simulink model "sim_notch440"  (R2021a)
settings: Solver=FixedStepDiscrete  StartTime=0.0  StopTime=3.9  FixedStep=6.25e-5  RelTol=1e-3
libraries: dspvision x1, simulink x1
settings Model: Creator=ricar  LastModifiedBy=rodri
settings SolverCC: AlgebraicLoopSolver=TrustRegion
settings DebuggingCC: SFMachineParentedDataDiag=warning

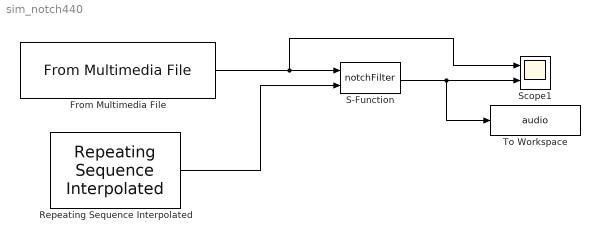
== system sim_notch440 ==
  From Multimedia File : dspvision/From Multimedia File  inputFilename=C:\Users\rodri\Desktop\Semestre_11\ELO314_Lab-DSP\Lab-DSP\lab3dsp_G6_Graves_Mardones\labC\sources\s-function_notch2\alternate_tones_16_16.wav  readRange=[1 Inf]  loop=on  numPlays=inf  outputStreams=Audio only  videoDataType=single  audioDataType=double  inheritSampleTime=on  userDefinedSampleTime=1/30  noAudioOutput=off  isIntensityVideo=off  fourcc=RGB  colorVideoFormat=Separate color signals  outputEOF=off  dataOrg=Column-major  audioFrameSize=1  computeAudioFrameSize=off  outSamplingMode=Sample based
  Repeating Sequence Interpolated : simulink/Sources/Repeating Sequence Interpolated  OutValues=[440 440 880 880].'  TimeValues=[0 1 3 4].'  LookUpMeth=Interpolation-Use End Values  tsamp=0.01  OutMin=[]  OutMax=[]  OutDataTypeStr=double  OutputDataTypeScalingMode=double  OutDataType=fixdt(0,8)  OutScaling=2^-10
  S-Function : S-Function  FunctionName=notchFilter  SFunctionDeploymentMode=off  EnableBusSupport=off
  Scope1 : Scope  NumInputPorts=2
  To Workspace : ToWorkspace  VariableName=audio  SampleTime=-1
  wires:
  S-Function/1 -> To Workspace/1, Scope1/2
  From Multimedia File/1 -> S-Function/1, Scope1/1
  Repeating Sequence Interpolated/1 -> S-Function/2
